simulink model "Pitch_attitude"  (R2024a)
settings: Solver=VariableStepAuto  StartTime=0.0  StopTime=50  RelTol=1e-3
model workspace (MAT data in the model file):
  At = 0.01309
libraries: simulink x2
settings Model: Creator=adamk  LastModifiedBy=adamk

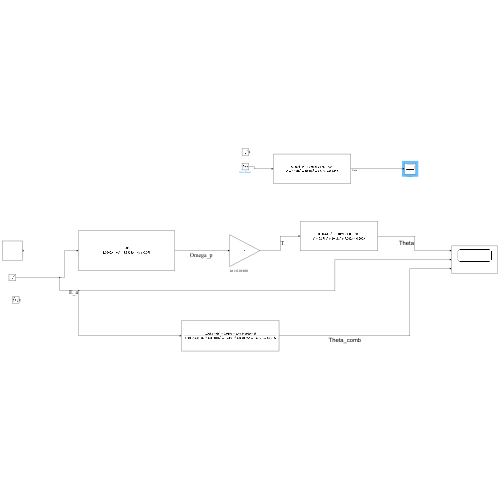
[thumbnail: Simulink's stored preview of the top-level diagram]
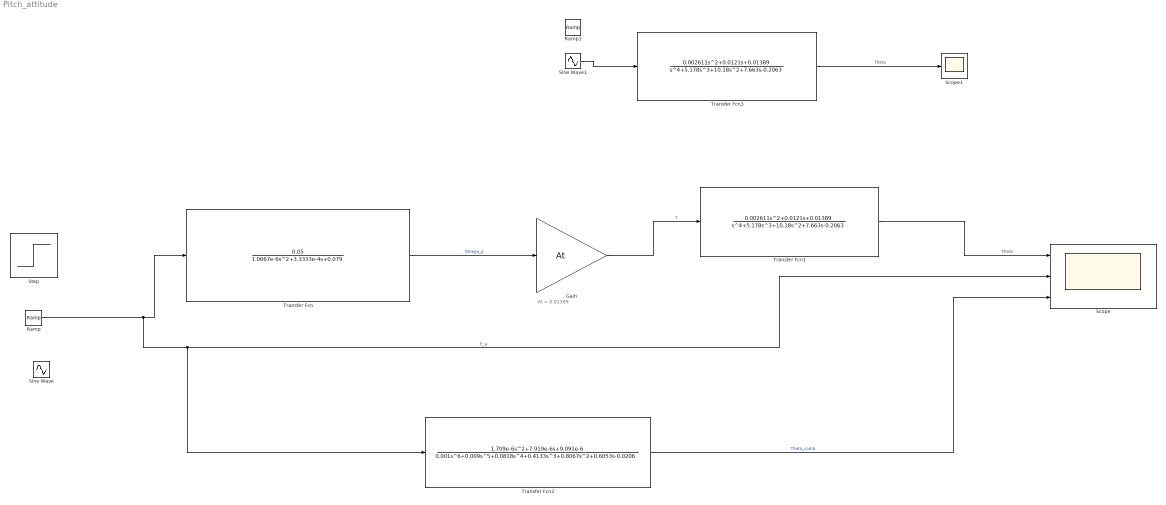
== system Pitch_attitude ==
  note: At = 0.01309
  Gain : Gain  Gain=At
  Ramp : simulink/Sources/Ramp  slope=50  start=0  InitialOutput=0
  Ramp1 : simulink/Sources/Ramp  slope=1  start=0  InitialOutput=0
  Scope : Scope  NumInputPorts=3
  Scope1 : Scope
  Sine Wave : Sin  SampleTime=0
  Sine Wave1 : Sin  SampleTime=0
  Step : Step  SampleTime=0
  Transfer Fcn : TransferFcn  Numerator=[0.05]  Denominator=[1.0667e-6 3.3333e-4 0.079]
  Transfer Fcn1 : TransferFcn  Numerator=[0.002611 0.0121 0.01389]  Denominator=[1 5.178 10.18 7.663 -0.2063]
  Transfer Fcn2 : TransferFcn  Numerator=[1.709e-6 7.919e-6 9.091e-6]  Denominator=[0.001 0.009 0.0818 0.4133 0.8067 0.6053 -0.0206]
  Transfer Fcn3 : TransferFcn  Numerator=[0.002611 0.0121 0.01389]  Denominator=[1 5.178 10.18 7.663 -0.2063]
  wires:
  Ramp/1 -> Transfer Fcn2/1, Scope/2, Transfer Fcn/1  "E_a"
  Transfer Fcn/1 -> Gain/1  "Omega_p"
  Gain/1 -> Transfer Fcn1/1  "T"
  Transfer Fcn1/1 -> Scope/1  "Theta"
  Transfer Fcn2/1 -> Scope/3  "Theta_comb"
  Transfer Fcn3/1 -> Scope1/1  "Theta"
  Sine Wave1/1 -> Transfer Fcn3/1
